simulink model "canLogPlayerModel"  (R2018a)
settings: Solver=FixedStepDiscrete  StartTime=0.0  StopTime=50000  RelTol=1e-3  EnableMultiTasking=on
undefined symbols (not defined in the file or in its folder): canChannel
libraries: simulink x30, canmsglib x15, canlib x3
(part 1 of 2)
settings Model: FPTRunName=Active  Creator=The MathWorks, Inc.  LastModifiedBy=Giovanni
settings DataIOCC: LimitDataPoints=on  SaveFormat=Array
settings OptimizationCC: BlockReduction=off  ExpressionDepthLimit=2147483647  LifeSpan=inf
settings DebuggingCC: UnderspecifiedInitializationDetection=Classic  MergeDetectMultiDrivingBlocksExec=none  SolverPrmCheckMsg=warning  FcnCallInpInsideContextMsg=warning  StateNameClashWarn=warning  SFUnexpectedBacktrackingDiag=warning  SFNoUnconditionalDefaultTransitionDiag=warning  SFExecutionAtInitializationDiag=none
settings HardwareCC: ProdBitPerPointer=32  ProdBitPerSizeT=32  ProdBitPerPtrDiffT=32  ProdLargestAtomicFloat=None  ProdIntDivRoundTo=Undefined  ProdEndianess=Unspecified  ProdWordSize=32  ProdHWDeviceType=32-bit Generic
settings ModelReferenceCC: PropagateSignalLabelsOutOfModel=off
settings RTWCC: PostCodeGenCommand=packNGo(buildInfo)  Description=Generic Real-Time Target  RetainRTWFile=on  TLCDebug=on
settings CodeAppCC: StateflowObjectComments=on
settings GRTTargetCC: TargetLangStandard=C89/C90 (ANSI)  GeneratePreprocessorConditionals=Disable all  CombineOutputUpdateFcns=off  MatFileLogging=off  GRTInterface=on
settings ConfigComp: CovMetricSettings=dw  CovHtmlReporting=on  CovSaveCumulativeToWorkspaceVar=on  CovSaveSingleToWorkspaceVar=on  CovExternalEMLEnable=off

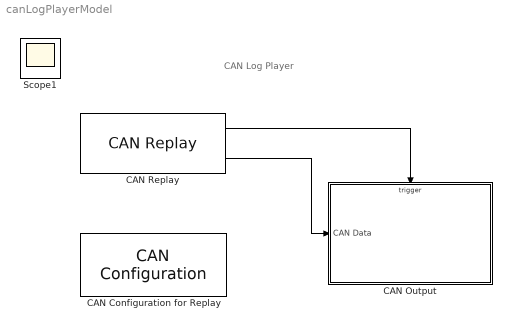
== system canLogPlayerModel ==
  note: CAN Log Player
  CAN Configuration for Replay : canlib/CAN Configuration  BlockHandle=5.0001  DeviceMenu=MathWorks Virtual 1 (Channel 1)  Device=MathWorks Virtual 1 (Channel 1)  ObjConstructor=canChannel('MathWorks', 'Virtual 1', 1)  BusSpeed=500000  EnableBitParameters=off  SJW=0  TSEG1=0  TSEG2=0  NSamples=0  AckMode=Normal
      settings: SourceProductName=Vehicle Network Toolbox  SourceProductBaseCode=VN
  CAN Output : Subsystem  TreatAsAtomicUnit=on
      settings: RTWSystemCode=Nonreusable function
  CAN Replay : canlib/CAN Replay  BlockHandle=121.0002  FullPathFileName=C:\Users\Giovanni\Documents\MATLAB\Maserati\CAN Log Player\log_0703_radars_replay.mat  FileName=log_0703_radars_replay.mat  VariableName=canMsgs  NoTimesReplay=Inf  ReplayTo=Output port  DeviceMenu=Select a device  Device=Select a device  ObjConstructor=Select a constructor  SampleTime=0.01  BusOutput=off
      settings: SourceProductName=Vehicle Network Toolbox  SourceProductBaseCode=VN
  Scope1 : Scope
  wires:
  CAN Replay/2 -> CAN Output/1(CAN Data)
  CAN Replay/1 -> CAN Output/Trigger

== system canLogPlayerModel/CAN Output ==
  CAN Data : Inport
  function : TriggerPort  TriggerType=function-call  VariantControl=Variant
  CAN Log : canlib/CAN Log  Commented=on  BlockHandle=9.0001  FullPathFileName=outputLog.mat  FileName=outputLog.mat  VariableName=outMsgs  MaxNumMessages=100000  LogFrom=Input port  DeviceMenu=Select a device  Device=Select a device  ObjConstructor=Select a constructor  SampleTime=0.01
      settings: SourceProductName=Vehicle Network Toolbox  SourceProductBaseCode=VN
  Command Sensors 1-4 : Subsystem  VariantControl=Variant1
  Sync : Subsystem
  Targets 0-9 : Subsystem
  wires:
  CAN Data/1 -> CAN Log/1, Sync/1(CAN data), Targets 0-9/1(In1), Command Sensors 1-4/1(CAN Data)

== system canLogPlayerModel/CAN Output/Command Sensors 1-4 ==
  CAN Data : Inport
  CAN Unpack Command : Subsystem
  Display Command 4 : Display
      settings: Format=hex (Stored Integer)
  Mux : Mux
  wires:
  CAN Data/1 -> CAN Unpack Command/1(In1)
  CAN Unpack Command/1(Command 1) -> Mux/1
  CAN Unpack Command/2(Command 2) -> Mux/2
  CAN Unpack Command/3(Command 3) -> Mux/3
  CAN Unpack Command/4(Command 4) -> Mux/4
  Mux/1 -> Display Command 4/1

== system canLogPlayerModel/CAN Output/Sync ==
  CAN data : Inport
  CAN Unpack Sync : canmsglib/CAN Unpack  CANdbFile=VehicleInfo.dbc  MsgList=WheelSpeeds  MsgName=Sync  MsgIDType=Standard (11-bit identifier)  MsgIdentifier=hex2dec('100')  MsgLength=8  SignalInfo=LF_WSpeed$8$16$2$2$1$0$1.000000e-02$-100$0$2000$#LR_WSpeed$40$16$2$2$1$0$1.000000e-02$-100$0$2000$#RF_WSpeed$24$16$2$2$1$0$1.000000e-02$-100$0$2000$#RR_WSpeed$56$16$2$2$1$0$1.000000e-02$-100$0$2000$#  NSignals=4  IDPort=off  TimestampPort=off  ErrorPort=off  RemotePort=off  LengthPort=off  StatusPort=off  StartBits=str2num('[int32(8);int32(40);int32(24);int32(56)]')  SignalSizes=str2num('[int32(16);int32(16);int32(16);int32(16)]')  ByteOrders=str2num('[int32(2);int32(2);int32(2);int32(2)]')  DataTypes=str2num('[int32(2);int32(2);int32(2);int32(2)]')  MultiplexTypes=str2num('[int32(1);int32(1);int32(1);int32(1)]')  MultiplexValues=str2num('[double(0);double(0);double(0);double(0)]')  Factors=str2num('[double(1.000000e-02);double(1.000000e-02);double(1.000000e-02);double(1.000000e-02)]')  Offsets=str2num('[double(-100);double(-100);double(-100);double(-100)]')  Minimums=str2num('[double(0);double(0);double(0);double(0)]')  Maximums=str2num('[double(2000);double(2000);double(2000);double(2000)]')  ApplyMinMax=off
      settings: SourceProductName=Simulink Real-Time  SourceProductBaseCode=XP  DataFormat=raw data
  Display Sync : Display
      settings: Format=hex (Stored Integer)
  wires:
  CAN Unpack Sync/1 -> Display Sync/1
  CAN data/1 -> CAN Unpack Sync/1

== system canLogPlayerModel/CAN Output/Targets 0-9 ==
  In1 : Inport
  CAN Unpack Target : Subsystem
  Display Targets : Display
      settings: Format=hex (Stored Integer)
  Mux : Mux  Inputs=10
  Subsystem : Subsystem
  wires:
  In1/1 -> CAN Unpack Target/1(In1)
  Mux/1 -> Display Targets/1
  CAN Unpack Target/3(Target 2) -> Mux/3, Subsystem/3(CAN Target 2)
  CAN Unpack Target/4(Target 3) -> Mux/4, Subsystem/4(CAN Target 3)
  CAN Unpack Target/5(Target 4) -> Mux/5, Subsystem/5(CAN Target 4)
  CAN Unpack Target/6(Target 5) -> Mux/6, Subsystem/6(CAN Target 5)
  CAN Unpack Target/7(Target 6) -> Mux/7, Subsystem/7(CAN Target 6)
  CAN Unpack Target/8(Target 7) -> Mux/8, Subsystem/8(CAN Target 7)
  CAN Unpack Target/9(Target 8) -> Mux/9, Subsystem/9(CAN Target 8)
  CAN Unpack Target/10(Target 9) -> Mux/10, Subsystem/10(CAN Target 9)
  CAN Unpack Target/1(Target 0) -> Mux/1, Subsystem/1(CAN Target 0)
  CAN Unpack Target/2(Target 1) -> Mux/2, Subsystem/2(CAN Target 1)

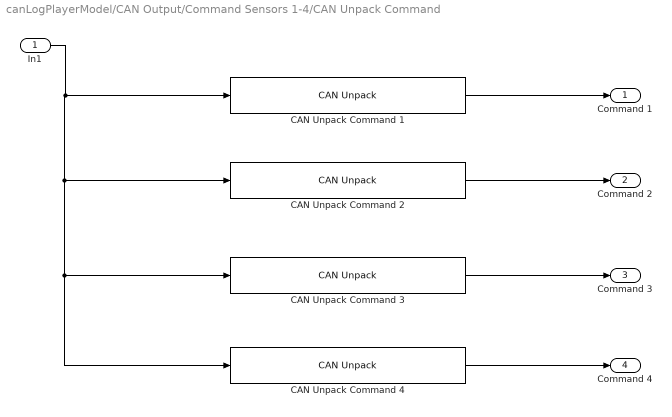
== system canLogPlayerModel/CAN Output/Command Sensors 1-4/CAN Unpack Command ==
  In1 : Inport
  CAN Unpack Command 1 : canmsglib/CAN Unpack  CANdbFile=VehicleInfo.dbc  MsgList=WheelSpeeds  MsgName=Command 1  MsgIDType=Standard (11-bit identifier)  MsgIdentifier=hex2dec('201')  MsgLength=8  SignalInfo=LF_WSpeed$8$16$2$2$1$0$1.000000e-02$-100$0$2000$#LR_WSpeed$40$16$2$2$1$0$1.000000e-02$-100$0$2000$#RF_WSpeed$24$16$2$2$1$0$1.000000e-02$-100$0$2000$#RR_WSpeed$56$16$2$2$1$0$1.000000e-02$-100$0$2000$#  NSignals=4  IDPort=off  TimestampPort=off  ErrorPort=off  RemotePort=off  LengthPort=off  StatusPort=off  StartBits=str2num('[int32(8);int32(40);int32(24);int32(56)]')  SignalSizes=str2num('[int32(16);int32(16);int32(16);int32(16)]')  ByteOrders=str2num('[int32(2);int32(2);int32(2);int32(2)]')  DataTypes=str2num('[int32(2);int32(2);int32(2);int32(2)]')  MultiplexTypes=str2num('[int32(1);int32(1);int32(1);int32(1)]')  MultiplexValues=str2num('[double(0);double(0);double(0);double(0)]')  Factors=str2num('[double(1.000000e-02);double(1.000000e-02);double(1.000000e-02);double(1.000000e-02)]')  Offsets=str2num('[double(-100);double(-100);double(-100);double(-100)]')  Minimums=str2num('[double(0);double(0);double(0);double(0)]')  Maximums=str2num('[double(2000);double(2000);double(2000);double(2000)]')  ApplyMinMax=off
      settings: SourceProductName=Simulink Real-Time  SourceProductBaseCode=XP  DataFormat=raw data
  CAN Unpack Command 2 : canmsglib/CAN Unpack  CANdbFile=VehicleInfo.dbc  MsgList=WheelSpeeds  MsgName=Command 2  MsgIDType=Standard (11-bit identifier)  MsgIdentifier=hex2dec('202')  MsgLength=8  SignalInfo=LF_WSpeed$8$16$2$2$1$0$1.000000e-02$-100$0$2000$#LR_WSpeed$40$16$2$2$1$0$1.000000e-02$-100$0$2000$#RF_WSpeed$24$16$2$2$1$0$1.000000e-02$-100$0$2000$#RR_WSpeed$56$16$2$2$1$0$1.000000e-02$-100$0$2000$#  NSignals=4  IDPort=off  TimestampPort=off  ErrorPort=off  RemotePort=off  LengthPort=off  StatusPort=off  StartBits=str2num('[int32(8);int32(40);int32(24);int32(56)]')  SignalSizes=str2num('[int32(16);int32(16);int32(16);int32(16)]')  ByteOrders=str2num('[int32(2);int32(2);int32(2);int32(2)]')  DataTypes=str2num('[int32(2);int32(2);int32(2);int32(2)]')  MultiplexTypes=str2num('[int32(1);int32(1);int32(1);int32(1)]')  MultiplexValues=str2num('[double(0);double(0);double(0);double(0)]')  Factors=str2num('[double(1.000000e-02);double(1.000000e-02);double(1.000000e-02);double(1.000000e-02)]')  Offsets=str2num('[double(-100);double(-100);double(-100);double(-100)]')  Minimums=str2num('[double(0);double(0);double(0);double(0)]')  Maximums=str2num('[double(2000);double(2000);double(2000);double(2000)]')  ApplyMinMax=off
      settings: SourceProductName=Simulink Real-Time  SourceProductBaseCode=XP  DataFormat=raw data
  CAN Unpack Command 3 : canmsglib/CAN Unpack  CANdbFile=VehicleInfo.dbc  MsgList=WheelSpeeds  MsgName=Command 3  MsgIDType=Standard (11-bit identifier)  MsgIdentifier=hex2dec('203')  MsgLength=8  SignalInfo=LF_WSpeed$8$16$2$2$1$0$1.000000e-02$-100$0$2000$#LR_WSpeed$40$16$2$2$1$0$1.000000e-02$-100$0$2000$#RF_WSpeed$24$16$2$2$1$0$1.000000e-02$-100$0$2000$#RR_WSpeed$56$16$2$2$1$0$1.000000e-02$-100$0$2000$#  NSignals=4  IDPort=off  TimestampPort=off  ErrorPort=off  RemotePort=off  LengthPort=off  StatusPort=off  StartBits=str2num('[int32(8);int32(40);int32(24);int32(56)]')  SignalSizes=str2num('[int32(16);int32(16);int32(16);int32(16)]')  ByteOrders=str2num('[int32(2);int32(2);int32(2);int32(2)]')  DataTypes=str2num('[int32(2);int32(2);int32(2);int32(2)]')  MultiplexTypes=str2num('[int32(1);int32(1);int32(1);int32(1)]')  MultiplexValues=str2num('[double(0);double(0);double(0);double(0)]')  Factors=str2num('[double(1.000000e-02);double(1.000000e-02);double(1.000000e-02);double(1.000000e-02)]')  Offsets=str2num('[double(-100);double(-100);double(-100);double(-100)]')  Minimums=str2num('[double(0);double(0);double(0);double(0)]')  Maximums=str2num('[double(2000);double(2000);double(2000);double(2000)]')  ApplyMinMax=off
      settings: SourceProductName=Simulink Real-Time  SourceProductBaseCode=XP  DataFormat=raw data
  CAN Unpack Command 4 : canmsglib/CAN Unpack  CANdbFile=VehicleInfo.dbc  MsgList=WheelSpeeds  MsgName=Command 4  MsgIDType=Standard (11-bit identifier)  MsgIdentifier=hex2dec('204')  MsgLength=8  SignalInfo=LF_WSpeed$8$16$2$2$1$0$1.000000e-02$-100$0$2000$#LR_WSpeed$40$16$2$2$1$0$1.000000e-02$-100$0$2000$#RF_WSpeed$24$16$2$2$1$0$1.000000e-02$-100$0$2000$#RR_WSpeed$56$16$2$2$1$0$1.000000e-02$-100$0$2000$#  NSignals=4  IDPort=off  TimestampPort=off  ErrorPort=off  RemotePort=off  LengthPort=off  StatusPort=off  StartBits=str2num('[int32(8);int32(40);int32(24);int32(56)]')  SignalSizes=str2num('[int32(16);int32(16);int32(16);int32(16)]')  ByteOrders=str2num('[int32(2);int32(2);int32(2);int32(2)]')  DataTypes=str2num('[int32(2);int32(2);int32(2);int32(2)]')  MultiplexTypes=str2num('[int32(1);int32(1);int32(1);int32(1)]')  MultiplexValues=str2num('[double(0);double(0);double(0);double(0)]')  Factors=str2num('[double(1.000000e-02);double(1.000000e-02);double(1.000000e-02);double(1.000000e-02)]')  Offsets=str2num('[double(-100);double(-100);double(-100);double(-100)]')  Minimums=str2num('[double(0);double(0);double(0);double(0)]')  Maximums=str2num('[double(2000);double(2000);double(2000);double(2000)]')  ApplyMinMax=off
      settings: SourceProductName=Simulink Real-Time  SourceProductBaseCode=XP  DataFormat=raw data
  Command 1 : Outport
  Command 2 : Outport  Port=2
  Command 3 : Outport  Port=3
  Command 4 : Outport  Port=4
  wires:
  In1/1 -> CAN Unpack Command 1/1, CAN Unpack Command 4/1, CAN Unpack Command 3/1, CAN Unpack Command 2/1
  CAN Unpack Command 4/1 -> Command 4/1
  CAN Unpack Command 2/1 -> Command 2/1
  CAN Unpack Command 3/1 -> Command 3/1
  CAN Unpack Command 1/1 -> Command 1/1

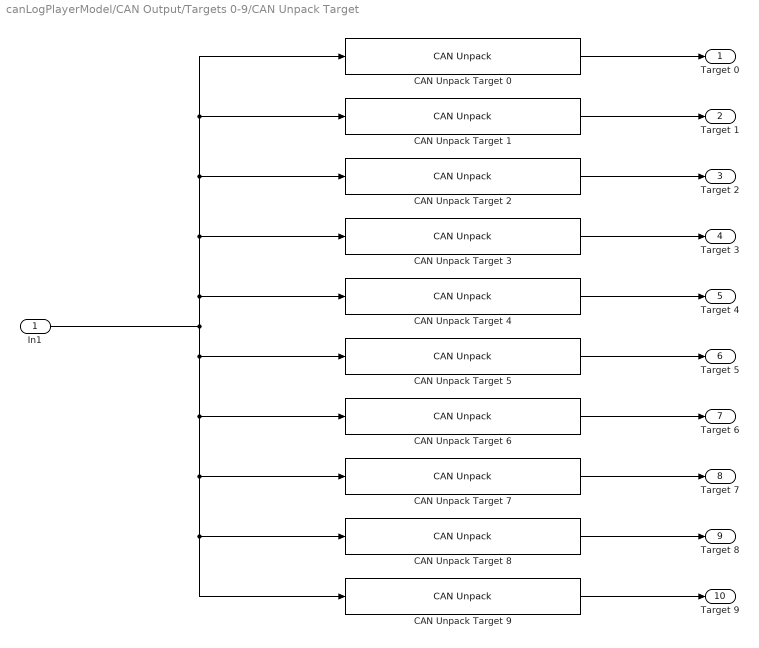
== system canLogPlayerModel/CAN Output/Targets 0-9/CAN Unpack Target ==
  In1 : Inport
  CAN Unpack Target 0 : canmsglib/CAN Unpack  CANdbFile=VehicleInfo.dbc  MsgList=WheelSpeeds  MsgName=Target 0  MsgIDType=Standard (11-bit identifier)  MsgIdentifier=hex2dec('300')  MsgLength=8  SignalInfo=LF_WSpeed$8$16$2$2$1$0$1.000000e-02$-100$0$2000$#LR_WSpeed$40$16$2$2$1$0$1.000000e-02$-100$0$2000$#RF_WSpeed$24$16$2$2$1$0$1.000000e-02$-100$0$2000$#RR_WSpeed$56$16$2$2$1$0$1.000000e-02$-100$0$2000$#  NSignals=4  IDPort=off  TimestampPort=off  ErrorPort=off  RemotePort=off  LengthPort=off  StatusPort=off  StartBits=str2num('[int32(8);int32(40);int32(24);int32(56)]')  SignalSizes=str2num('[int32(16);int32(16);int32(16);int32(16)]')  ByteOrders=str2num('[int32(2);int32(2);int32(2);int32(2)]')  DataTypes=str2num('[int32(2);int32(2);int32(2);int32(2)]')  MultiplexTypes=str2num('[int32(1);int32(1);int32(1);int32(1)]')  MultiplexValues=str2num('[double(0);double(0);double(0);double(0)]')  Factors=str2num('[double(1.000000e-02);double(1.000000e-02);double(1.000000e-02);double(1.000000e-02)]')  Offsets=str2num('[double(-100);double(-100);double(-100);double(-100)]')  Minimums=str2num('[double(0);double(0);double(0);double(0)]')  Maximums=str2num('[double(2000);double(2000);double(2000);double(2000)]')  ApplyMinMax=off
      settings: SourceProductName=Simulink Real-Time  SourceProductBaseCode=XP  DataFormat=raw data
  CAN Unpack Target 1 : canmsglib/CAN Unpack  CANdbFile=VehicleInfo.dbc  MsgList=WheelSpeeds  MsgName=Target 1  MsgIDType=Standard (11-bit identifier)  MsgIdentifier=hex2dec('301')  MsgLength=8  SignalInfo=LF_WSpeed$8$16$2$2$1$0$1.000000e-02$-100$0$2000$#LR_WSpeed$40$16$2$2$1$0$1.000000e-02$-100$0$2000$#RF_WSpeed$24$16$2$2$1$0$1.000000e-02$-100$0$2000$#RR_WSpeed$56$16$2$2$1$0$1.000000e-02$-100$0$2000$#  NSignals=4  IDPort=off  TimestampPort=off  ErrorPort=off  RemotePort=off  LengthPort=off  StatusPort=off  StartBits=str2num('[int32(8);int32(40);int32(24);int32(56)]')  SignalSizes=str2num('[int32(16);int32(16);int32(16);int32(16)]')  ByteOrders=str2num('[int32(2);int32(2);int32(2);int32(2)]')  DataTypes=str2num('[int32(2);int32(2);int32(2);int32(2)]')  MultiplexTypes=str2num('[int32(1);int32(1);int32(1);int32(1)]')  MultiplexValues=str2num('[double(0);double(0);double(0);double(0)]')  Factors=str2num('[double(1.000000e-02);double(1.000000e-02);double(1.000000e-02);double(1.000000e-02)]')  Offsets=str2num('[double(-100);double(-100);double(-100);double(-100)]')  Minimums=str2num('[double(0);double(0);double(0);double(0)]')  Maximums=str2num('[double(2000);double(2000);double(2000);double(2000)]')  ApplyMinMax=off
      settings: SourceProductName=Simulink Real-Time  SourceProductBaseCode=XP  DataFormat=raw data
  CAN Unpack Target 2 : canmsglib/CAN Unpack  CANdbFile=VehicleInfo.dbc  MsgList=WheelSpeeds  MsgName=Target 2  MsgIDType=Standard (11-bit identifier)  MsgIdentifier=hex2dec('302')  MsgLength=8  SignalInfo=LF_WSpeed$8$16$2$2$1$0$1.000000e-02$-100$0$2000$#LR_WSpeed$40$16$2$2$1$0$1.000000e-02$-100$0$2000$#RF_WSpeed$24$16$2$2$1$0$1.000000e-02$-100$0$2000$#RR_WSpeed$56$16$2$2$1$0$1.000000e-02$-100$0$2000$#  NSignals=4  IDPort=off  TimestampPort=off  ErrorPort=off  RemotePort=off  LengthPort=off  StatusPort=off  StartBits=str2num('[int32(8);int32(40);int32(24);int32(56)]')  SignalSizes=str2num('[int32(16);int32(16);int32(16);int32(16)]')  ByteOrders=str2num('[int32(2);int32(2);int32(2);int32(2)]')  DataTypes=str2num('[int32(2);int32(2);int32(2);int32(2)]')  MultiplexTypes=str2num('[int32(1);int32(1);int32(1);int32(1)]')  MultiplexValues=str2num('[double(0);double(0);double(0);double(0)]')  Factors=str2num('[double(1.000000e-02);double(1.000000e-02);double(1.000000e-02);double(1.000000e-02)]')  Offsets=str2num('[double(-100);double(-100);double(-100);double(-100)]')  Minimums=str2num('[double(0);double(0);double(0);double(0)]')  Maximums=str2num('[double(2000);double(2000);double(2000);double(2000)]')  ApplyMinMax=off
      settings: SourceProductName=Simulink Real-Time  SourceProductBaseCode=XP  DataFormat=raw data
  CAN Unpack Target 3 : canmsglib/CAN Unpack  CANdbFile=VehicleInfo.dbc  MsgList=WheelSpeeds  MsgName=Target 3  MsgIDType=Standard (11-bit identifier)  MsgIdentifier=hex2dec('303')  MsgLength=8  SignalInfo=LF_WSpeed$8$16$2$2$1$0$1.000000e-02$-100$0$2000$#LR_WSpeed$40$16$2$2$1$0$1.000000e-02$-100$0$2000$#RF_WSpeed$24$16$2$2$1$0$1.000000e-02$-100$0$2000$#RR_WSpeed$56$16$2$2$1$0$1.000000e-02$-100$0$2000$#  NSignals=4  IDPort=off  TimestampPort=off  ErrorPort=off  RemotePort=off  LengthPort=off  StatusPort=off  StartBits=str2num('[int32(8);int32(40);int32(24);int32(56)]')  SignalSizes=str2num('[int32(16);int32(16);int32(16);int32(16)]')  ByteOrders=str2num('[int32(2);int32(2);int32(2);int32(2)]')  DataTypes=str2num('[int32(2);int32(2);int32(2);int32(2)]')  MultiplexTypes=str2num('[int32(1);int32(1);int32(1);int32(1)]')  MultiplexValues=str2num('[double(0);double(0);double(0);double(0)]')  Factors=str2num('[double(1.000000e-02);double(1.000000e-02);double(1.000000e-02);double(1.000000e-02)]')  Offsets=str2num('[double(-100);double(-100);double(-100);double(-100)]')  Minimums=str2num('[double(0);double(0);double(0);double(0)]')  Maximums=str2num('[double(2000);double(2000);double(2000);double(2000)]')  ApplyMinMax=off
      settings: SourceProductName=Simulink Real-Time  SourceProductBaseCode=XP  DataFormat=raw data
  CAN Unpack Target 4 : canmsglib/CAN Unpack  CANdbFile=VehicleInfo.dbc  MsgList=WheelSpeeds  MsgName=Target 4  MsgIDType=Standard (11-bit identifier)  MsgIdentifier=hex2dec('304')  MsgLength=8  SignalInfo=LF_WSpeed$8$16$2$2$1$0$1.000000e-02$-100$0$2000$#LR_WSpeed$40$16$2$2$1$0$1.000000e-02$-100$0$2000$#RF_WSpeed$24$16$2$2$1$0$1.000000e-02$-100$0$2000$#RR_WSpeed$56$16$2$2$1$0$1.000000e-02$-100$0$2000$#  NSignals=4  IDPort=off  TimestampPort=off  ErrorPort=off  RemotePort=off  LengthPort=off  StatusPort=off  StartBits=str2num('[int32(8);int32(40);int32(24);int32(56)]')  SignalSizes=str2num('[int32(16);int32(16);int32(16);int32(16)]')  ByteOrders=str2num('[int32(2);int32(2);int32(2);int32(2)]')  DataTypes=str2num('[int32(2);int32(2);int32(2);int32(2)]')  MultiplexTypes=str2num('[int32(1);int32(1);int32(1);int32(1)]')  MultiplexValues=str2num('[double(0);double(0);double(0);double(0)]')  Factors=str2num('[double(1.000000e-02);double(1.000000e-02);double(1.000000e-02);double(1.000000e-02)]')  Offsets=str2num('[double(-100);double(-100);double(-100);double(-100)]')  Minimums=str2num('[double(0);double(0);double(0);double(0)]')  Maximums=str2num('[double(2000);double(2000);double(2000);double(2000)]')  ApplyMinMax=off
      settings: SourceProductName=Simulink Real-Time  SourceProductBaseCode=XP  DataFormat=raw data
  CAN Unpack Target 5 : canmsglib/CAN Unpack  CANdbFile=VehicleInfo.dbc  MsgList=WheelSpeeds  MsgName=Target 5  MsgIDType=Standard (11-bit identifier)  MsgIdentifier=hex2dec('305')  MsgLength=8  SignalInfo=LF_WSpeed$8$16$2$2$1$0$1.000000e-02$-100$0$2000$#LR_WSpeed$40$16$2$2$1$0$1.000000e-02$-100$0$2000$#RF_WSpeed$24$16$2$2$1$0$1.000000e-02$-100$0$2000$#RR_WSpeed$56$16$2$2$1$0$1.000000e-02$-100$0$2000$#  NSignals=4  IDPort=off  TimestampPort=off  ErrorPort=off  RemotePort=off  LengthPort=off  StatusPort=off  StartBits=str2num('[int32(8);int32(40);int32(24);int32(56)]')  SignalSizes=str2num('[int32(16);int32(16);int32(16);int32(16)]')  ByteOrders=str2num('[int32(2);int32(2);int32(2);int32(2)]')  DataTypes=str2num('[int32(2);int32(2);int32(2);int32(2)]')  MultiplexTypes=str2num('[int32(1);int32(1);int32(1);int32(1)]')  MultiplexValues=str2num('[double(0);double(0);double(0);double(0)]')  Factors=str2num('[double(1.000000e-02);double(1.000000e-02);double(1.000000e-02);double(1.000000e-02)]')  Offsets=str2num('[double(-100);double(-100);double(-100);double(-100)]')  Minimums=str2num('[double(0);double(0);double(0);double(0)]')  Maximums=str2num('[double(2000);double(2000);double(2000);double(2000)]')  ApplyMinMax=off
      settings: SourceProductName=Simulink Real-Time  SourceProductBaseCode=XP  DataFormat=raw data
  CAN Unpack Target 6 : canmsglib/CAN Unpack  CANdbFile=VehicleInfo.dbc  MsgList=WheelSpeeds  MsgName=Target 6  MsgIDType=Standard (11-bit identifier)  MsgIdentifier=hex2dec('306')  MsgLength=8  SignalInfo=LF_WSpeed$8$16$2$2$1$0$1.000000e-02$-100$0$2000$#LR_WSpeed$40$16$2$2$1$0$1.000000e-02$-100$0$2000$#RF_WSpeed$24$16$2$2$1$0$1.000000e-02$-100$0$2000$#RR_WSpeed$56$16$2$2$1$0$1.000000e-02$-100$0$2000$#  NSignals=4  IDPort=off  TimestampPort=off  ErrorPort=off  RemotePort=off  LengthPort=off  StatusPort=off  StartBits=str2num('[int32(8);int32(40);int32(24);int32(56)]')  SignalSizes=str2num('[int32(16);int32(16);int32(16);int32(16)]')  ByteOrders=str2num('[int32(2);int32(2);int32(2);int32(2)]')  DataTypes=str2num('[int32(2);int32(2);int32(2);int32(2)]')  MultiplexTypes=str2num('[int32(1);int32(1);int32(1);int32(1)]')  MultiplexValues=str2num('[double(0);double(0);double(0);double(0)]')  Factors=str2num('[double(1.000000e-02);double(1.000000e-02);double(1.000000e-02);double(1.000000e-02)]')  Offsets=str2num('[double(-100);double(-100);double(-100);double(-100)]')  Minimums=str2num('[double(0);double(0);double(0);double(0)]')  Maximums=str2num('[double(2000);double(2000);double(2000);double(2000)]')  ApplyMinMax=off
      settings: SourceProductName=Simulink Real-Time  SourceProductBaseCode=XP  DataFormat=raw data
  CAN Unpack Target 7 : canmsglib/CAN Unpack  CANdbFile=VehicleInfo.dbc  MsgList=WheelSpeeds  MsgName=Target 7  MsgIDType=Standard (11-bit identifier)  MsgIdentifier=hex2dec('307')  MsgLength=8  SignalInfo=LF_WSpeed$8$16$2$2$1$0$1.000000e-02$-100$0$2000$#LR_WSpeed$40$16$2$2$1$0$1.000000e-02$-100$0$2000$#RF_WSpeed$24$16$2$2$1$0$1.000000e-02$-100$0$2000$#RR_WSpeed$56$16$2$2$1$0$1.000000e-02$-100$0$2000$#  NSignals=4  IDPort=off  TimestampPort=off  ErrorPort=off  RemotePort=off  LengthPort=off  StatusPort=off  StartBits=str2num('[int32(8);int32(40);int32(24);int32(56)]')  SignalSizes=str2num('[int32(16);int32(16);int32(16);int32(16)]')  ByteOrders=str2num('[int32(2);int32(2);int32(2);int32(2)]')  DataTypes=str2num('[int32(2);int32(2);int32(2);int32(2)]')  MultiplexTypes=str2num('[int32(1);int32(1);int32(1);int32(1)]')  MultiplexValues=str2num('[double(0);double(0);double(0);double(0)]')  Factors=str2num('[double(1.000000e-02);double(1.000000e-02);double(1.000000e-02);double(1.000000e-02)]')  Offsets=str2num('[double(-100);double(-100);double(-100);double(-100)]')  Minimums=str2num('[double(0);double(0);double(0);double(0)]')  Maximums=str2num('[double(2000);double(2000);double(2000);double(2000)]')  ApplyMinMax=off
      settings: SourceProductName=Simulink Real-Time  SourceProductBaseCode=XP  DataFormat=raw data
  CAN Unpack Target 8 : canmsglib/CAN Unpack  CANdbFile=VehicleInfo.dbc  MsgList=WheelSpeeds  MsgName=Target 8  MsgIDType=Standard (11-bit identifier)  MsgIdentifier=hex2dec('308')  MsgLength=8  SignalInfo=LF_WSpeed$8$16$2$2$1$0$1.000000e-02$-100$0$2000$#LR_WSpeed$40$16$2$2$1$0$1.000000e-02$-100$0$2000$#RF_WSpeed$24$16$2$2$1$0$1.000000e-02$-100$0$2000$#RR_WSpeed$56$16$2$2$1$0$1.000000e-02$-100$0$2000$#  NSignals=4  IDPort=off  TimestampPort=off  ErrorPort=off  RemotePort=off  LengthPort=off  StatusPort=off  StartBits=str2num('[int32(8);int32(40);int32(24);int32(56)]')  SignalSizes=str2num('[int32(16);int32(16);int32(16);int32(16)]')  ByteOrders=str2num('[int32(2);int32(2);int32(2);int32(2)]')  DataTypes=str2num('[int32(2);int32(2);int32(2);int32(2)]')  MultiplexTypes=str2num('[int32(1);int32(1);int32(1);int32(1)]')  MultiplexValues=str2num('[double(0);double(0);double(0);double(0)]')  Factors=str2num('[double(1.000000e-02);double(1.000000e-02);double(1.000000e-02);double(1.000000e-02)]')  Offsets=str2num('[double(-100);double(-100);double(-100);double(-100)]')  Minimums=str2num('[double(0);double(0);double(0);double(0)]')  Maximums=str2num('[double(2000);double(2000);double(2000);double(2000)]')  ApplyMinMax=off
      settings: SourceProductName=Simulink Real-Time  SourceProductBaseCode=XP  DataFormat=raw data
  CAN Unpack Target 9 : canmsglib/CAN Unpack  CANdbFile=VehicleInfo.dbc  MsgList=WheelSpeeds  MsgName=Target 9  MsgIDType=Standard (11-bit identifier)  MsgIdentifier=hex2dec('309')  MsgLength=8  SignalInfo=LF_WSpeed$8$16$2$2$1$0$1.000000e-02$-100$0$2000$#LR_WSpeed$40$16$2$2$1$0$1.000000e-02$-100$0$2000$#RF_WSpeed$24$16$2$2$1$0$1.000000e-02$-100$0$2000$#RR_WSpeed$56$16$2$2$1$0$1.000000e-02$-100$0$2000$#  NSignals=4  IDPort=off  TimestampPort=off  ErrorPort=off  RemotePort=off  LengthPort=off  StatusPort=off  StartBits=str2num('[int32(8);int32(40);int32(24);int32(56)]')  SignalSizes=str2num('[int32(16);int32(16);int32(16);int32(16)]')  ByteOrders=str2num('[int32(2);int32(2);int32(2);int32(2)]')  DataTypes=str2num('[int32(2);int32(2);int32(2);int32(2)]')  MultiplexTypes=str2num('[int32(1);int32(1);int32(1);int32(1)]')  MultiplexValues=str2num('[double(0);double(0);double(0);double(0)]')  Factors=str2num('[double(1.000000e-02);double(1.000000e-02);double(1.000000e-02);double(1.000000e-02)]')  Offsets=str2num('[double(-100);double(-100);double(-100);double(-100)]')  Minimums=str2num('[double(0);double(0);double(0);double(0)]')  Maximums=str2num('[double(2000);double(2000);double(2000);double(2000)]')  ApplyMinMax=off
      settings: SourceProductName=Simulink Real-Time  SourceProductBaseCode=XP  DataFormat=raw data
  Target 0 : Outport
  Target 1 : Outport  Port=2
  Target 2 : Outport  Port=3
  Target 3 : Outport  Port=4
  Target 4 : Outport  Port=5
  Target 5 : Outport  Port=6
  Target 6 : Outport  Port=7
  Target 7 : Outport  Port=8
  Target 8 : Outport  Port=9
  Target 9 : Outport  Port=10
  wires:
  In1/1 -> CAN Unpack Target 0/1, CAN Unpack Target 1/1, CAN Unpack Target 2/1, CAN Unpack Target 3/1, CAN Unpack Target 4/1, CAN Unpack Target 9/1, CAN Unpack Target 8/1, CAN Unpack Target 7/1, CAN Unpack Target 6/1, CAN Unpack Target 5/1
  CAN Unpack Target 3/1 -> Target 3/1
  CAN Unpack Target 8/1 -> Target 8/1
  CAN Unpack Target 2/1 -> Target 2/1
  CAN Unpack Target 1/1 -> Target 1/1
  CAN Unpack Target 4/1 -> Target 4/1
  CAN Unpack Target 5/1 -> Target 5/1
  CAN Unpack Target 7/1 -> Target 7/1
  CAN Unpack Target 6/1 -> Target 6/1
  CAN Unpack Target 0/1 -> Target 0/1
  CAN Unpack Target 9/1 -> Target 9/1

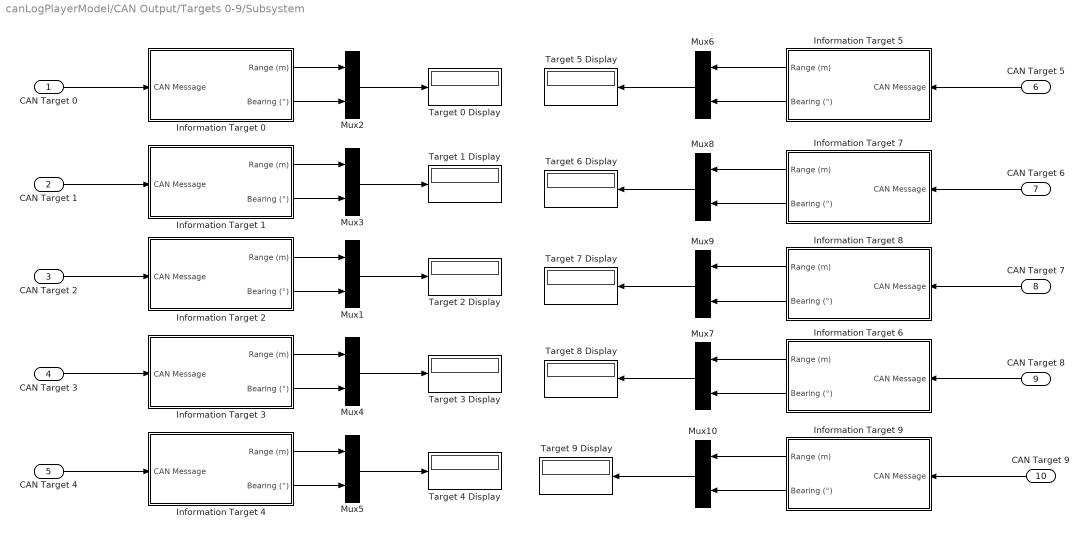
== system canLogPlayerModel/CAN Output/Targets 0-9/Subsystem ==
  CAN Target 0 : Inport
  CAN Target 1 : Inport  Port=2
  CAN Target 2 : Inport  Port=3
  CAN Target 3 : Inport  Port=4
  CAN Target 4 : Inport  Port=5
  CAN Target 5 : Inport  Port=6
  CAN Target 6 : Inport  Port=7
  CAN Target 7 : Inport  Port=8
  CAN Target 8 : Inport  Port=9
  CAN Target 9 : Inport  Port=10
  Information Target 0 : Subsystem
  Information Target 1 : Subsystem
  Information Target 2 : Subsystem
  Information Target 3 : Subsystem
  Information Target 4 : Subsystem
  Information Target 5 : Subsystem
  Information Target 6 : Subsystem
  Information Target 7 : Subsystem
  Information Target 8 : Subsystem
  Information Target 9 : Subsystem
  Mux{1..10} (10 alike) : Mux  Inputs=2
  Target 0 Display : Display
  Target 1 Display : Display
  Target 2 Display : Display
  Target 3 Display : Display
  Target 4 Display : Display
  Target 5 Display : Display
  Target 6 Display : Display
  Target 7 Display : Display
  Target 8 Display : Display
  Target 9 Display : Display
  wires:
  Information Target 4/2(Bearing (°)) -> Mux5/2
  Mux5/1 -> Target 4 Display/1
  Information Target 8/2(Bearing (°)) -> Mux9/2
  Mux4/1 -> Target 3 Display/1
  Information Target 0/2(Bearing (°)) -> Mux2/2
  Information Target 0/1(Range (m)) -> Mux2/1
  Information Target 3/2(Bearing (°)) -> Mux4/2
  Information Target 2/2(Bearing (°)) -> Mux1/2
  Information Target 4/1(Range (m)) -> Mux5/1
  Information Target 7/1(Range (m)) -> Mux8/1
  Information Target 3/1(Range (m)) -> Mux4/1
  Information Target 1/1(Range (m)) -> Mux3/1
  CAN Target 5/1 -> Information Target 5/1(CAN Message)
  CAN Target 1/1 -> Information Target 1/1(CAN Message)
  Mux3/1 -> Target 1 Display/1
  Information Target 1/2(Bearing (°)) -> Mux3/2
  CAN Target 0/1 -> Information Target 0/1(CAN Message)
  Mux2/1 -> Target 0 Display/1
  CAN Target 2/1 -> Information Target 2/1(CAN Message)
  Information Target 2/1(Range (m)) -> Mux1/1
  CAN Target 3/1 -> Information Target 3/1(CAN Message)
  Mux1/1 -> Target 2 Display/1
  Mux9/1 -> Target 7 Display/1
  Mux8/1 -> Target 6 Display/1
  Information Target 5/1(Range (m)) -> Mux6/1
  Mux7/1 -> Target 8 Display/1
  Information Target 6/1(Range (m)) -> Mux7/1
  Information Target 6/2(Bearing (°)) -> Mux7/2
  CAN Target 4/1 -> Information Target 4/1(CAN Message)
  Information Target 8/1(Range (m)) -> Mux9/1
  Information Target 9/1(Range (m)) -> Mux10/1
  Mux10/1 -> Target 9 Display/1
  Information Target 7/2(Bearing (°)) -> Mux8/2
  Mux6/1 -> Target 5 Display/1
  CAN Target 8/1 -> Information Target 6/1(CAN Message)
  Information Target 5/2(Bearing (°)) -> Mux6/2
  CAN Target 9/1 -> Information Target 9/1(CAN Message)
  CAN Target 6/1 -> Information Target 7/1(CAN Message)
  CAN Target 7/1 -> Information Target 8/1(CAN Message)
  Information Target 9/2(Bearing (°)) -> Mux10/2

== system canLogPlayerModel/CAN Output/Targets 0-9/Subsystem/Information Target 0 ==
  CAN Message : Inport
  Check Target Format : Subsystem
  Target Format 2 : Subsystem
  Terminator : Terminator
  Terminator1 : Terminator
  Range (m) : Outport
  Bearing (°) : Outport  Port=2
  wires:
  Target Format 2/2(Bearing (°)) -> Bearing (°)/1
  Check Target Format/1(Is format 1?) -> Terminator/1
  CAN Message/1 -> Check Target Format/1(CAN Message), Target Format 2/1(CAN Message)
  Check Target Format/2(Is format 2?) -> Target Format 2/Enable
  Check Target Format/3(Is format 3?) -> Terminator1/1
  Target Format 2/1(Range (m)) -> Range (m)/1

== system canLogPlayerModel/CAN Output/Targets 0-9/Subsystem/Information Target 1 ==
  CAN Message : Inport
  Check Target Format : Subsystem
  Target Format 2 : Subsystem
  Terminator : Terminator
  Terminator1 : Terminator
  Range (m) : Outport
  Bearing (°) : Outport  Port=2
  wires:
  Target Format 2/2(Bearing (°)) -> Bearing (°)/1
  Check Target Format/1(Is format 1?) -> Terminator/1
  CAN Message/1 -> Check Target Format/1(CAN Message), Target Format 2/1(CAN Message)
  Check Target Format/2(Is format 2?) -> Target Format 2/Enable
  Check Target Format/3(Is format 3?) -> Terminator1/1
  Target Format 2/1(Range (m)) -> Range (m)/1

== system canLogPlayerModel/CAN Output/Targets 0-9/Subsystem/Information Target 2 ==
  CAN Message : Inport
  Check Target Format : Subsystem
  Target Format 2 : Subsystem
  Terminator : Terminator
  Terminator1 : Terminator
  Range (m) : Outport
  Bearing (°) : Outport  Port=2
  wires:
  Target Format 2/2(Bearing (°)) -> Bearing (°)/1
  Check Target Format/1(Is format 1?) -> Terminator/1
  CAN Message/1 -> Check Target Format/1(CAN Message), Target Format 2/1(CAN Message)
  Check Target Format/2(Is format 2?) -> Target Format 2/Enable
  Check Target Format/3(Is format 3?) -> Terminator1/1
  Target Format 2/1(Range (m)) -> Range (m)/1

== system canLogPlayerModel/CAN Output/Targets 0-9/Subsystem/Information Target 3 ==
  CAN Message : Inport
  Check Target Format : Subsystem
  Target Format 2 : Subsystem
  Terminator : Terminator
  Terminator1 : Terminator
  Range (m) : Outport
  Bearing (°) : Outport  Port=2
  wires:
  Target Format 2/2(Bearing (°)) -> Bearing (°)/1
  Check Target Format/1(Is format 1?) -> Terminator/1
  CAN Message/1 -> Check Target Format/1(CAN Message), Target Format 2/1(CAN Message)
  Check Target Format/2(Is format 2?) -> Target Format 2/Enable
  Check Target Format/3(Is format 3?) -> Terminator1/1
  Target Format 2/1(Range (m)) -> Range (m)/1

== system canLogPlayerModel/CAN Output/Targets 0-9/Subsystem/Information Target 4 ==
  CAN Message : Inport
  Check Target Format : Subsystem
  Target Format 2 : Subsystem
  Terminator : Terminator
  Terminator1 : Terminator
  Range (m) : Outport
  Bearing (°) : Outport  Port=2
  wires:
  Target Format 2/2(Bearing (°)) -> Bearing (°)/1
  Check Target Format/1(Is format 1?) -> Terminator/1
  CAN Message/1 -> Check Target Format/1(CAN Message), Target Format 2/1(CAN Message)
  Check Target Format/2(Is format 2?) -> Target Format 2/Enable
  Check Target Format/3(Is format 3?) -> Terminator1/1
  Target Format 2/1(Range (m)) -> Range (m)/1

== system canLogPlayerModel/CAN Output/Targets 0-9/Subsystem/Information Target 5 ==
  CAN Message : Inport
  Check Target Format : Subsystem
  Target Format 2 : Subsystem
  Terminator : Terminator
  Terminator1 : Terminator
  Range (m) : Outport
  Bearing (°) : Outport  Port=2
  wires:
  Target Format 2/2(Bearing (°)) -> Bearing (°)/1
  Check Target Format/1(Is format 1?) -> Terminator/1
  CAN Message/1 -> Check Target Format/1(CAN Message), Target Format 2/1(CAN Message)
  Check Target Format/2(Is format 2?) -> Target Format 2/Enable
  Check Target Format/3(Is format 3?) -> Terminator1/1
  Target Format 2/1(Range (m)) -> Range (m)/1

== system canLogPlayerModel/CAN Output/Targets 0-9/Subsystem/Information Target 6 ==
  CAN Message : Inport
  Check Target Format : Subsystem
  Target Format 2 : Subsystem
  Terminator : Terminator
  Terminator1 : Terminator
  Range (m) : Outport
  Bearing (°) : Outport  Port=2
  wires:
  Target Format 2/2(Bearing (°)) -> Bearing (°)/1
  Check Target Format/1(Is format 1?) -> Terminator/1
  CAN Message/1 -> Check Target Format/1(CAN Message), Target Format 2/1(CAN Message)
  Check Target Format/2(Is format 2?) -> Target Format 2/Enable
  Check Target Format/3(Is format 3?) -> Terminator1/1
  Target Format 2/1(Range (m)) -> Range (m)/1

== system canLogPlayerModel/CAN Output/Targets 0-9/Subsystem/Information Target 7 ==
  CAN Message : Inport
  Check Target Format : Subsystem
  Target Format 2 : Subsystem
  Terminator : Terminator
  Terminator1 : Terminator
  Range (m) : Outport
  Bearing (°) : Outport  Port=2
  wires:
  Target Format 2/2(Bearing (°)) -> Bearing (°)/1
  Check Target Format/1(Is format 1?) -> Terminator/1
  CAN Message/1 -> Check Target Format/1(CAN Message), Target Format 2/1(CAN Message)
  Check Target Format/2(Is format 2?) -> Target Format 2/Enable
  Check Target Format/3(Is format 3?) -> Terminator1/1
  Target Format 2/1(Range (m)) -> Range (m)/1

== system canLogPlayerModel/CAN Output/Targets 0-9/Subsystem/Information Target 8 ==
  CAN Message : Inport
  Check Target Format : Subsystem
  Target Format 2 : Subsystem
  Terminator : Terminator
  Terminator1 : Terminator
  Range (m) : Outport
  Bearing (°) : Outport  Port=2
  wires:
  Target Format 2/2(Bearing (°)) -> Bearing (°)/1
  Check Target Format/1(Is format 1?) -> Terminator/1
  CAN Message/1 -> Check Target Format/1(CAN Message), Target Format 2/1(CAN Message)
  Check Target Format/2(Is format 2?) -> Target Format 2/Enable
  Check Target Format/3(Is format 3?) -> Terminator1/1
  Target Format 2/1(Range (m)) -> Range (m)/1

== system canLogPlayerModel/CAN Output/Targets 0-9/Subsystem/Information Target 9 ==
  CAN Message : Inport
  Check Target Format : Subsystem
  Target Format 2 : Subsystem
  Terminator : Terminator
  Terminator1 : Terminator
  Range (m) : Outport
  Bearing (°) : Outport  Port=2
  wires:
  Target Format 2/2(Bearing (°)) -> Bearing (°)/1
  Check Target Format/1(Is format 1?) -> Terminator/1
  CAN Message/1 -> Check Target Format/1(CAN Message), Target Format 2/1(CAN Message)
  Check Target Format/2(Is format 2?) -> Target Format 2/Enable
  Check Target Format/3(Is format 3?) -> Terminator1/1
  Target Format 2/1(Range (m)) -> Range (m)/1

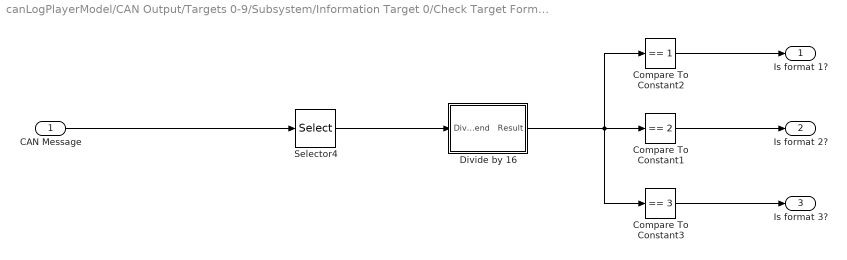
== system canLogPlayerModel/CAN Output/Targets 0-9/Subsystem/Information Target 0/Check Target Format ==
  CAN Message : Inport
  Compare To Constant1 : simulink/Logic and Bit Operations/Compare To Constant  relop===  const=2  OutDataTypeStr=boolean
  Compare To Constant2 : simulink/Logic and Bit Operations/Compare To Constant  relop===  const=1  OutDataTypeStr=boolean
  Compare To Constant3 : simulink/Logic and Bit Operations/Compare To Constant  relop===  const=3  OutDataTypeStr=boolean
  Divide by 16 : Subsystem
  Selector4 : Selector  IndexMode=Zero-based  InputPortWidth=8  IndexOptions=Index vector (dialog)  Indices=6  OutputSizes=1
  Is format 1? : Outport
  Is format 2? : Outport  Port=2
  Is format 3? : Outport  Port=3
  wires:
  Divide by 16/1(Result) -> Compare To Constant3/1, Compare To Constant2/1, Compare To Constant1/1
  CAN Message/1 -> Selector4/1
  Selector4/1 -> Divide by 16/1(Dividend)
  Compare To Constant1/1 -> Is format 2?/1
  Compare To Constant2/1 -> Is format 1?/1
  Compare To Constant3/1 -> Is format 3?/1

== system canLogPlayerModel/CAN Output/Targets 0-9/Subsystem/Information Target 0/Target Format 2 ==
  CAN Message : Inport
  Enable : EnablePort
  Bearing : Subsystem
  Range : Subsystem
  Range (m) : Outport
  Bearing (°) : Outport  Port=2
  wires:
  CAN Message/1 -> Bearing/1(CAN Message), Range/1(CAN Message)
  Range/1(Range (m)) -> Range (m)/1
  Bearing/1(Bearing (°)) -> Bearing (°)/1

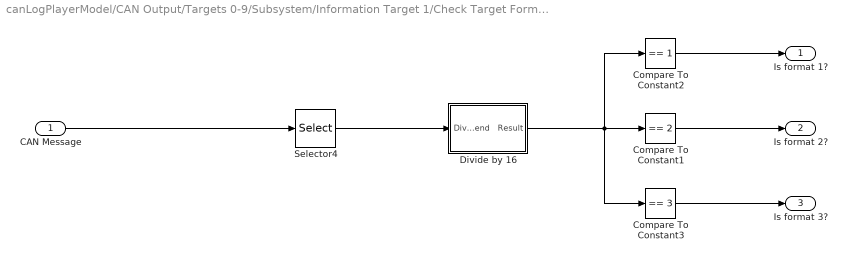
== system canLogPlayerModel/CAN Output/Targets 0-9/Subsystem/Information Target 1/Check Target Format ==
  CAN Message : Inport
  Compare To Constant1 : simulink/Logic and Bit Operations/Compare To Constant  relop===  const=2  OutDataTypeStr=boolean
  Compare To Constant2 : simulink/Logic and Bit Operations/Compare To Constant  relop===  const=1  OutDataTypeStr=boolean
  Compare To Constant3 : simulink/Logic and Bit Operations/Compare To Constant  relop===  const=3  OutDataTypeStr=boolean
  Divide by 16 : Subsystem
  Selector4 : Selector  IndexMode=Zero-based  InputPortWidth=8  IndexOptions=Index vector (dialog)  Indices=6  OutputSizes=1
  Is format 1? : Outport
  Is format 2? : Outport  Port=2
  Is format 3? : Outport  Port=3
  wires:
  Divide by 16/1(Result) -> Compare To Constant3/1, Compare To Constant2/1, Compare To Constant1/1
  CAN Message/1 -> Selector4/1
  Selector4/1 -> Divide by 16/1(Dividend)
  Compare To Constant1/1 -> Is format 2?/1
  Compare To Constant2/1 -> Is format 1?/1
  Compare To Constant3/1 -> Is format 3?/1

== system canLogPlayerModel/CAN Output/Targets 0-9/Subsystem/Information Target 1/Target Format 2 ==
  CAN Message : Inport
  Enable : EnablePort
  Bearing : Subsystem
  Range : Subsystem
  Range (m) : Outport
  Bearing (°) : Outport  Port=2
  wires:
  CAN Message/1 -> Bearing/1(CAN Message), Range/1(CAN Message)
  Range/1(Range (m)) -> Range (m)/1
  Bearing/1(Bearing (°)) -> Bearing (°)/1

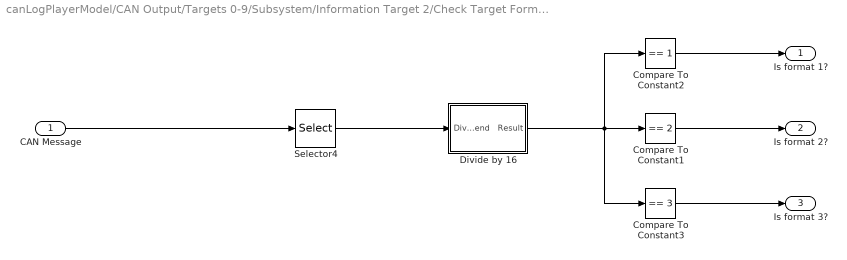
== system canLogPlayerModel/CAN Output/Targets 0-9/Subsystem/Information Target 2/Check Target Format ==
  CAN Message : Inport
  Compare To Constant1 : simulink/Logic and Bit Operations/Compare To Constant  relop===  const=2  OutDataTypeStr=boolean
  Compare To Constant2 : simulink/Logic and Bit Operations/Compare To Constant  relop===  const=1  OutDataTypeStr=boolean
  Compare To Constant3 : simulink/Logic and Bit Operations/Compare To Constant  relop===  const=3  OutDataTypeStr=boolean
  Divide by 16 : Subsystem
  Selector4 : Selector  IndexMode=Zero-based  InputPortWidth=8  IndexOptions=Index vector (dialog)  Indices=6  OutputSizes=1
  Is format 1? : Outport
  Is format 2? : Outport  Port=2
  Is format 3? : Outport  Port=3
  wires:
  Divide by 16/1(Result) -> Compare To Constant3/1, Compare To Constant2/1, Compare To Constant1/1
  CAN Message/1 -> Selector4/1
  Selector4/1 -> Divide by 16/1(Dividend)
  Compare To Constant1/1 -> Is format 2?/1
  Compare To Constant2/1 -> Is format 1?/1
  Compare To Constant3/1 -> Is format 3?/1

== system canLogPlayerModel/CAN Output/Targets 0-9/Subsystem/Information Target 2/Target Format 2 ==
  CAN Message : Inport
  Enable : EnablePort
  Bearing : Subsystem
  Range : Subsystem
  Range (m) : Outport
  Bearing (°) : Outport  Port=2
  wires:
  CAN Message/1 -> Bearing/1(CAN Message), Range/1(CAN Message)
  Range/1(Range (m)) -> Range (m)/1
  Bearing/1(Bearing (°)) -> Bearing (°)/1

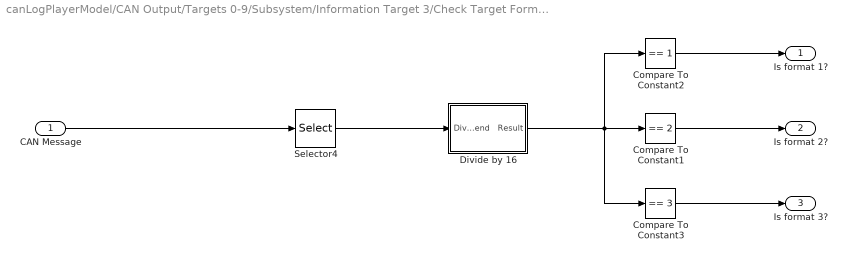
== system canLogPlayerModel/CAN Output/Targets 0-9/Subsystem/Information Target 3/Check Target Format ==
  CAN Message : Inport
  Compare To Constant1 : simulink/Logic and Bit Operations/Compare To Constant  relop===  const=2  OutDataTypeStr=boolean
  Compare To Constant2 : simulink/Logic and Bit Operations/Compare To Constant  relop===  const=1  OutDataTypeStr=boolean
  Compare To Constant3 : simulink/Logic and Bit Operations/Compare To Constant  relop===  const=3  OutDataTypeStr=boolean
  Divide by 16 : Subsystem
  Selector4 : Selector  IndexMode=Zero-based  InputPortWidth=8  IndexOptions=Index vector (dialog)  Indices=6  OutputSizes=1
  Is format 1? : Outport
  Is format 2? : Outport  Port=2
  Is format 3? : Outport  Port=3
  wires:
  Divide by 16/1(Result) -> Compare To Constant3/1, Compare To Constant2/1, Compare To Constant1/1
  CAN Message/1 -> Selector4/1
  Selector4/1 -> Divide by 16/1(Dividend)
  Compare To Constant1/1 -> Is format 2?/1
  Compare To Constant2/1 -> Is format 1?/1
  Compare To Constant3/1 -> Is format 3?/1

== system canLogPlayerModel/CAN Output/Targets 0-9/Subsystem/Information Target 3/Target Format 2 ==
  CAN Message : Inport
  Enable : EnablePort
  Bearing : Subsystem
  Range : Subsystem
  Range (m) : Outport
  Bearing (°) : Outport  Port=2
  wires:
  CAN Message/1 -> Bearing/1(CAN Message), Range/1(CAN Message)
  Range/1(Range (m)) -> Range (m)/1
  Bearing/1(Bearing (°)) -> Bearing (°)/1

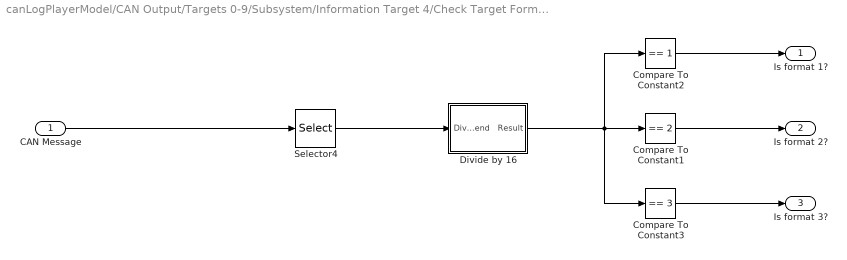
== system canLogPlayerModel/CAN Output/Targets 0-9/Subsystem/Information Target 4/Check Target Format ==
  CAN Message : Inport
  Compare To Constant1 : simulink/Logic and Bit Operations/Compare To Constant  relop===  const=2  OutDataTypeStr=boolean
  Compare To Constant2 : simulink/Logic and Bit Operations/Compare To Constant  relop===  const=1  OutDataTypeStr=boolean
  Compare To Constant3 : simulink/Logic and Bit Operations/Compare To Constant  relop===  const=3  OutDataTypeStr=boolean
  Divide by 16 : Subsystem
  Selector4 : Selector  IndexMode=Zero-based  InputPortWidth=8  IndexOptions=Index vector (dialog)  Indices=6  OutputSizes=1
  Is format 1? : Outport
  Is format 2? : Outport  Port=2
  Is format 3? : Outport  Port=3
  wires:
  Divide by 16/1(Result) -> Compare To Constant3/1, Compare To Constant2/1, Compare To Constant1/1
  CAN Message/1 -> Selector4/1
  Selector4/1 -> Divide by 16/1(Dividend)
  Compare To Constant1/1 -> Is format 2?/1
  Compare To Constant2/1 -> Is format 1?/1
  Compare To Constant3/1 -> Is format 3?/1

== system canLogPlayerModel/CAN Output/Targets 0-9/Subsystem/Information Target 4/Target Format 2 ==
  CAN Message : Inport
  Enable : EnablePort
  Bearing : Subsystem
  Range : Subsystem
  Range (m) : Outport
  Bearing (°) : Outport  Port=2
  wires:
  CAN Message/1 -> Bearing/1(CAN Message), Range/1(CAN Message)
  Range/1(Range (m)) -> Range (m)/1
  Bearing/1(Bearing (°)) -> Bearing (°)/1

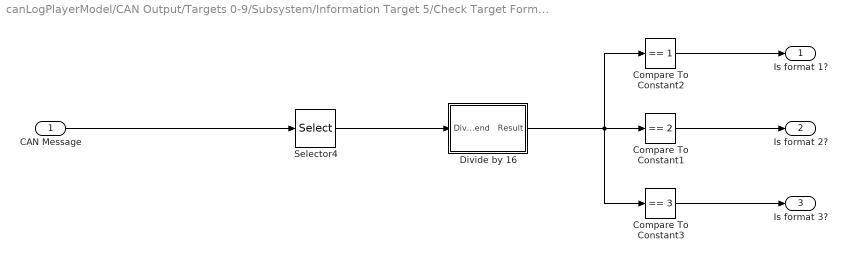
== system canLogPlayerModel/CAN Output/Targets 0-9/Subsystem/Information Target 5/Check Target Format ==
  CAN Message : Inport
  Compare To Constant1 : simulink/Logic and Bit Operations/Compare To Constant  relop===  const=2  OutDataTypeStr=boolean
  Compare To Constant2 : simulink/Logic and Bit Operations/Compare To Constant  relop===  const=1  OutDataTypeStr=boolean
  Compare To Constant3 : simulink/Logic and Bit Operations/Compare To Constant  relop===  const=3  OutDataTypeStr=boolean
  Divide by 16 : Subsystem
  Selector4 : Selector  IndexMode=Zero-based  InputPortWidth=8  IndexOptions=Index vector (dialog)  Indices=6  OutputSizes=1
  Is format 1? : Outport
  Is format 2? : Outport  Port=2
  Is format 3? : Outport  Port=3
  wires:
  Divide by 16/1(Result) -> Compare To Constant3/1, Compare To Constant2/1, Compare To Constant1/1
  CAN Message/1 -> Selector4/1
  Selector4/1 -> Divide by 16/1(Dividend)
  Compare To Constant1/1 -> Is format 2?/1
  Compare To Constant2/1 -> Is format 1?/1
  Compare To Constant3/1 -> Is format 3?/1

== system canLogPlayerModel/CAN Output/Targets 0-9/Subsystem/Information Target 5/Target Format 2 ==
  CAN Message : Inport
  Enable : EnablePort
  Bearing : Subsystem
  Range : Subsystem
  Range (m) : Outport
  Bearing (°) : Outport  Port=2
  wires:
  CAN Message/1 -> Bearing/1(CAN Message), Range/1(CAN Message)
  Range/1(Range (m)) -> Range (m)/1
  Bearing/1(Bearing (°)) -> Bearing (°)/1

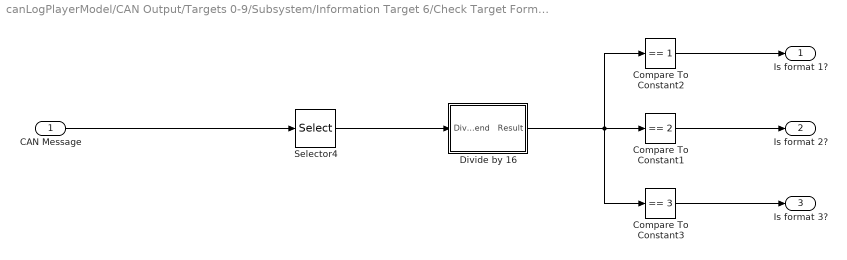
== system canLogPlayerModel/CAN Output/Targets 0-9/Subsystem/Information Target 6/Check Target Format ==
  CAN Message : Inport
  Compare To Constant1 : simulink/Logic and Bit Operations/Compare To Constant  relop===  const=2  OutDataTypeStr=boolean
  Compare To Constant2 : simulink/Logic and Bit Operations/Compare To Constant  relop===  const=1  OutDataTypeStr=boolean
  Compare To Constant3 : simulink/Logic and Bit Operations/Compare To Constant  relop===  const=3  OutDataTypeStr=boolean
  Divide by 16 : Subsystem
  Selector4 : Selector  IndexMode=Zero-based  InputPortWidth=8  IndexOptions=Index vector (dialog)  Indices=6  OutputSizes=1
  Is format 1? : Outport
  Is format 2? : Outport  Port=2
  Is format 3? : Outport  Port=3
  wires:
  Divide by 16/1(Result) -> Compare To Constant3/1, Compare To Constant2/1, Compare To Constant1/1
  CAN Message/1 -> Selector4/1
  Selector4/1 -> Divide by 16/1(Dividend)
  Compare To Constant1/1 -> Is format 2?/1
  Compare To Constant2/1 -> Is format 1?/1
  Compare To Constant3/1 -> Is format 3?/1

== system canLogPlayerModel/CAN Output/Targets 0-9/Subsystem/Information Target 6/Target Format 2 ==
  CAN Message : Inport
  Enable : EnablePort
  Bearing : Subsystem
  Range : Subsystem
  Range (m) : Outport
  Bearing (°) : Outport  Port=2
  wires:
  CAN Message/1 -> Bearing/1(CAN Message), Range/1(CAN Message)
  Range/1(Range (m)) -> Range (m)/1
  Bearing/1(Bearing (°)) -> Bearing (°)/1

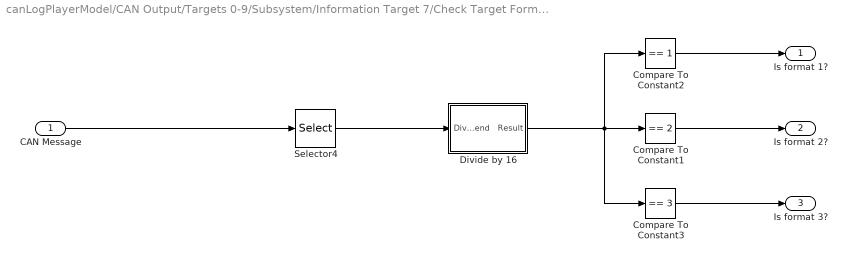
== system canLogPlayerModel/CAN Output/Targets 0-9/Subsystem/Information Target 7/Check Target Format ==
  CAN Message : Inport
  Compare To Constant1 : simulink/Logic and Bit Operations/Compare To Constant  relop===  const=2  OutDataTypeStr=boolean
  Compare To Constant2 : simulink/Logic and Bit Operations/Compare To Constant  relop===  const=1  OutDataTypeStr=boolean
  Compare To Constant3 : simulink/Logic and Bit Operations/Compare To Constant  relop===  const=3  OutDataTypeStr=boolean
  Divide by 16 : Subsystem
  Selector4 : Selector  IndexMode=Zero-based  InputPortWidth=8  IndexOptions=Index vector (dialog)  Indices=6  OutputSizes=1
  Is format 1? : Outport
  Is format 2? : Outport  Port=2
  Is format 3? : Outport  Port=3
  wires:
  Divide by 16/1(Result) -> Compare To Constant3/1, Compare To Constant2/1, Compare To Constant1/1
  CAN Message/1 -> Selector4/1
  Selector4/1 -> Divide by 16/1(Dividend)
  Compare To Constant1/1 -> Is format 2?/1
  Compare To Constant2/1 -> Is format 1?/1
  Compare To Constant3/1 -> Is format 3?/1

== system canLogPlayerModel/CAN Output/Targets 0-9/Subsystem/Information Target 7/Target Format 2 ==
  CAN Message : Inport
  Enable : EnablePort
  Bearing : Subsystem
  Range : Subsystem
  Range (m) : Outport
  Bearing (°) : Outport  Port=2
  wires:
  CAN Message/1 -> Bearing/1(CAN Message), Range/1(CAN Message)
  Range/1(Range (m)) -> Range (m)/1
  Bearing/1(Bearing (°)) -> Bearing (°)/1

== system canLogPlayerModel/CAN Output/Targets 0-9/Subsystem/Information Target 8/Check Target Format ==
  CAN Message : Inport
  Compare To Constant1 : simulink/Logic and Bit Operations/Compare To Constant  relop===  const=2  OutDataTypeStr=boolean
  Compare To Constant2 : simulink/Logic and Bit Operations/Compare To Constant  relop===  const=1  OutDataTypeStr=boolean
  Compare To Constant3 : simulink/Logic and Bit Operations/Compare To Constant  relop===  const=3  OutDataTypeStr=boolean
  Divide by 16 : Subsystem
  Selector4 : Selector  IndexMode=Zero-based  InputPortWidth=8  IndexOptions=Index vector (dialog)  Indices=6  OutputSizes=1
  Is format 1? : Outport
  Is format 2? : Outport  Port=2
  Is format 3? : Outport  Port=3
  wires:
  Divide by 16/1(Result) -> Compare To Constant3/1, Compare To Constant2/1, Compare To Constant1/1
  CAN Message/1 -> Selector4/1
  Selector4/1 -> Divide by 16/1(Dividend)
  Compare To Constant1/1 -> Is format 2?/1
  Compare To Constant2/1 -> Is format 1?/1
  Compare To Constant3/1 -> Is format 3?/1

== system canLogPlayerModel/CAN Output/Targets 0-9/Subsystem/Information Target 8/Target Format 2 ==
  CAN Message : Inport
  Enable : EnablePort
  Bearing : Subsystem
  Range : Subsystem
  Range (m) : Outport
  Bearing (°) : Outport  Port=2
  wires:
  CAN Message/1 -> Bearing/1(CAN Message), Range/1(CAN Message)
  Range/1(Range (m)) -> Range (m)/1
  Bearing/1(Bearing (°)) -> Bearing (°)/1
